simulink model "dynamicModelTest"  (R2021a)
settings: Solver=VariableStepAuto  StartTime=0.0  StopTime=10.0  RelTol=1e-3
values from neighbouring files (symbols this model uses):
  f_c_x = 0    [assignment5_main.m]
  f_c_y = 0    [assignment5_main.m]
  f_c_z = 0    [assignment5_main.m]
  tau_c_x = 0    [assignment5_main.m]
  tau_c_y = 0    [assignment5_main.m]
  tau_c_z = 0    [assignment5_main.m]
settings Model: Creator=fabio  LastModifiedBy=fabio

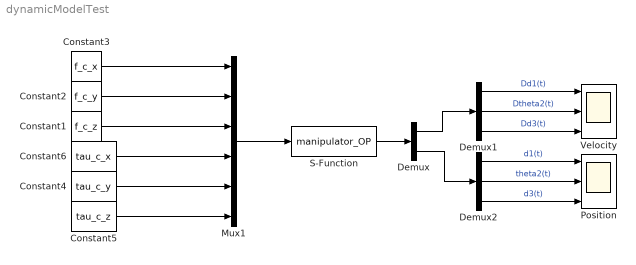
== system dynamicModelTest ==
  Constant1 : Constant  Value=f_c_z  VectorParams1D=off
  Constant2 : Constant  Value=f_c_y  VectorParams1D=off
  Constant3 : Constant  Value=f_c_x  VectorParams1D=off
  Constant4 : Constant  Value=tau_c_y  VectorParams1D=off
  Constant5 : Constant  Value=tau_c_z  VectorParams1D=off
  Constant6 : Constant  Value=tau_c_x  VectorParams1D=off
  Demux : Demux  Outputs=2
  Demux1 : Demux  Outputs=3
  Demux2 : Demux  Outputs=3
  Mux1 : Mux  Inputs=6
  Position : Scope  NumInputPorts=3
  S-Function : S-Function  FunctionName=manipulator_OP  Parameters=myRobot  SFunctionDeploymentMode=off  EnableBusSupport=off
  Velocity : Scope  NumInputPorts=3
  wires:
  Constant3/1 -> Mux1/1
  Constant2/1 -> Mux1/2
  Mux1/1 -> S-Function/1
  Demux/1 -> Demux1/1
  Demux1/1 -> Velocity/1  "Dd1(t)"
  Demux1/2 -> Velocity/2  "Dtheta2(t)"
  Demux1/3 -> Velocity/3  "Dd3(t)"
  Demux2/3 -> Position/3  "d3(t)"
  Demux2/2 -> Position/2  "theta2(t)"
  Demux2/1 -> Position/1  "d1(t)"
  Demux/2 -> Demux2/1
  S-Function/1 -> Demux/1
  Constant1/1 -> Mux1/3
  Constant6/1 -> Mux1/4
  Constant4/1 -> Mux1/5
  Constant5/1 -> Mux1/6
